simulink model "trigonometric_function"  (R2021a)
settings: Solver=VariableStepAuto  StartTime=0.0  StopTime=1  RelTol=1e-3
settings Model: Creator=Acer  LastModifiedBy=Acer

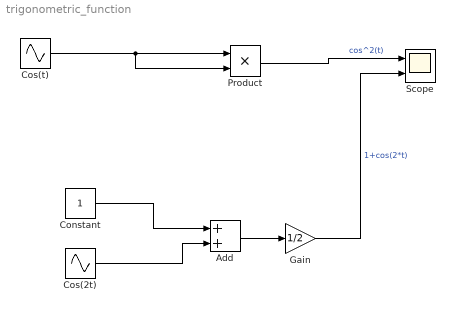
== system trigonometric_function ==
  Add : Sum
  Constant : Constant
  Cos(2t) : Sin  Frequency=2*pi*1*2  Phase=pi/2  SampleTime=0
  Cos(t) : Sin  Frequency=2*pi*1  Phase=pi/2  SampleTime=0
  Gain : Gain  Gain=1/2
  Product : Product
  Scope : Scope  NumInputPorts=2
  wires:
  Cos(t)/1 -> Product/2, Product/1
  Product/1 -> Scope/1  "cos^2(t)"
  Constant/1 -> Add/1
  Cos(2t)/1 -> Add/2
  Add/1 -> Gain/1
  Gain/1 -> Scope/2  "1+cos(2*t)"
